simulink model "Test_Bit_Demultiplexer_1_to_8"  (Simulink 8.1)
settings: Solver=ode45  StartTime=0.0  StopTime=len  RelTol=1e-3
libraries: commutil2 x3, Bit_Demultiplexers_Lib x1
settings Model: Creator=N  LastModifiedBy=uzivatel
settings DataIOCC: LimitDataPoints=off  SignalLoggingSaveFormat=Dataset
settings OptimizationCC: ExpressionDepthLimit=128
settings DebuggingCC: UnderspecifiedInitializationDetection=Simplified  MergeDetectMultiDrivingBlocksExec=error  SolverPrmCheckMsg=none  FcnCallInpInsideContextMsg=EnableAllAsError  FrameProcessingCompatibilityMsg=error  StateNameClashWarn=none
settings HardwareCC: ProdBitPerPointer=64  ProdLargestAtomicFloat=Float  ProdIntDivRoundTo=Zero  ProdEndianess=LittleEndian  ProdHWDeviceType=Intel->x86-64 (Windows64)
settings ModelReferenceCC: PropagateSignalLabelsOutOfModel=on
settings GRTTargetCC: CodeReplacementLibrary=None  CombineOutputUpdateFcns=on  CPPClassGenCompliant=on  GRTInterface=off

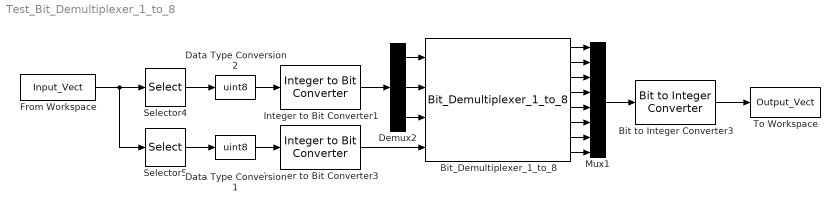
== system Test_Bit_Demultiplexer_1_to_8 ==
  Bit to Integer Converter3 : commutil2/Bit to Integer Converter  nbits=8  bitOrder=MSB first  signedOutputValues=Unsigned  outDtype=uint8  outDtypeSigned=Inherit via internal rule
  Bit_Demultiplexer_1_to_8 : Bit_Demultiplexers_Lib/Bit_Demultiplexers_Lib/Bit_Demultiplexer_1_to_8
  Data Type Conversion1 : DataTypeConversion  OutDataTypeStr=uint8
  Data Type Conversion2 : DataTypeConversion  OutDataTypeStr=uint8
  Demux2 : Demux  Outputs=3
  From Workspace : FromWorkspace  VariableName=Input_Vect  SampleTime=1  Interpolate=off  OutputAfterFinalValue=Holding final value
  Integer to Bit Converter1 : commutil2/Integer to Bit Converter  nbits=3  signedInputValues=Unsigned  bitOrder=MSB first  outDtype=uint8
  Integer to Bit Converter3 : commutil2/Integer to Bit Converter  nbits=1  signedInputValues=Unsigned  bitOrder=MSB first  outDtype=uint8
  Mux1 : Mux  Inputs=8
  Selector4 : Selector  IndexMode=Zero-based  InputPortWidth=2  SampleTime=1  IndexOptions=Index vector (dialog)  Indices=0  OutputSizes=1
  Selector5 : Selector  IndexMode=Zero-based  InputPortWidth=2  IndexOptions=Index vector (dialog)  Indices=1  OutputSizes=1
  To Workspace : ToWorkspace  VariableName=Output_Vect  SampleTime=1
  wires:
  Demux2/1 -> Bit_Demultiplexer_1_to_8/1
  Demux2/2 -> Bit_Demultiplexer_1_to_8/2
  Demux2/3 -> Bit_Demultiplexer_1_to_8/3
  Integer to Bit Converter1/1 -> Demux2/1
  Bit_Demultiplexer_1_to_8/1 -> Mux1/1
  Bit_Demultiplexer_1_to_8/8 -> Mux1/8
  Bit_Demultiplexer_1_to_8/2 -> Mux1/2
  Bit_Demultiplexer_1_to_8/3 -> Mux1/3
  Bit_Demultiplexer_1_to_8/4 -> Mux1/4
  Bit_Demultiplexer_1_to_8/5 -> Mux1/5
  Bit_Demultiplexer_1_to_8/6 -> Mux1/6
  Bit_Demultiplexer_1_to_8/7 -> Mux1/7
  Data Type Conversion2/1 -> Integer to Bit Converter1/1
  From Workspace/1 -> Selector5/1, Selector4/1
  Mux1/1 -> Bit to Integer Converter3/1
  Bit to Integer Converter3/1 -> To Workspace/1
  Selector4/1 -> Data Type Conversion2/1
  Selector5/1 -> Data Type Conversion1/1
  Data Type Conversion1/1 -> Integer to Bit Converter3/1
  Integer to Bit Converter3/1 -> Bit_Demultiplexer_1_to_8/4
